simulink model "fixpt_rounding_mode"  (R2015b)
settings: Solver=FixedStepDiscrete  SolverMode=SingleTasking  StartTime=0.0  StopTime=10  RelTol=1e-3
settings Model: Creator=amatsumo  LastModifiedBy=amatsumo
settings DataIOCC: SaveFormat=Array  SignalLoggingSaveFormat=ModelDataLogs  SaveOutput=off  SignalLogging=off  SaveTime=off
settings OptimizationCC: BlockReduction=off  ConditionallyExecuteInputs=off  DefaultParameterBehavior=Inlined  ExpressionDepthLimit=2147483647
settings DebuggingCC: AlgebraicLoopMsg=error  UnderspecifiedInitializationDetection=Classic  MergeDetectMultiDrivingBlocksExec=none  SolverPrmCheckMsg=warning  SingleTaskRateTransMsg=error  FcnCallInpInsideContextMsg=EnableAllAsWarning  StateNameClashWarn=warning
settings HardwareCC: ProdBitPerPointer=32  ProdLargestAtomicFloat=None  ProdIntDivRoundTo=Undefined  ProdEndianess=Unspecified  ProdWordSize=32  ProdHWDeviceType=ASIC/FPGA->ASIC/FPGA  ProdEqTarget=off
settings GRTTargetCC: GeneratePreprocessorConditionals=Disable all  CombineOutputUpdateFcns=off  GRTInterface=on
settings ConfigComp: CovModelRefEnable=Off  CovSFcnEnable=off

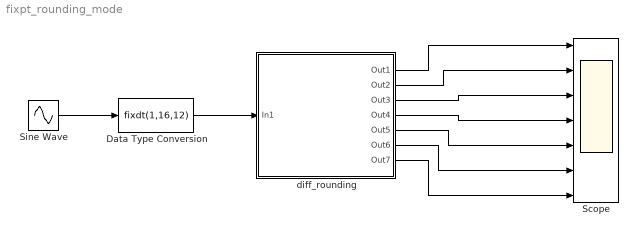
== system fixpt_rounding_mode ==
  Data Type Conversion : DataTypeConversion  OutDataTypeStr=fixdt(1,16,12)
  Scope : Scope  NumInputPorts=7
  Sine Wave : Sin  Frequency=2*pi*1  SampleTime=1/100
  diff_rounding : Subsystem
  wires:
  Sine Wave/1 -> Data Type Conversion/1
  Data Type Conversion/1 -> diff_rounding/1(In1)
  diff_rounding/1(Out1) -> Scope/1
  diff_rounding/2(Out2) -> Scope/2
  diff_rounding/3(Out3) -> Scope/3
  diff_rounding/4(Out4) -> Scope/4
  diff_rounding/5(Out5) -> Scope/5
  diff_rounding/6(Out6) -> Scope/6
  diff_rounding/7(Out7) -> Scope/7

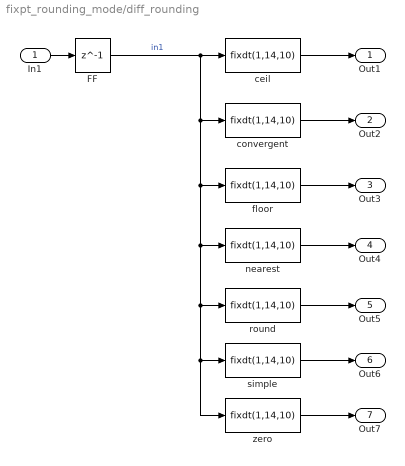
== system fixpt_rounding_mode/diff_rounding ==
  In1 : Inport
  FF : Delay  DelayLength=1
  ceil : DataTypeConversion  OutDataTypeStr=fixdt(1,14,10)  RndMeth=Ceiling
  convergent : DataTypeConversion  OutDataTypeStr=fixdt(1,14,10)  RndMeth=Convergent
  floor : DataTypeConversion  OutDataTypeStr=fixdt(1,14,10)
  nearest : DataTypeConversion  OutDataTypeStr=fixdt(1,14,10)  RndMeth=Nearest
  round : DataTypeConversion  OutDataTypeStr=fixdt(1,14,10)  RndMeth=Round
  simple : DataTypeConversion  OutDataTypeStr=fixdt(1,14,10)  RndMeth=Simplest
  zero : DataTypeConversion  OutDataTypeStr=fixdt(1,14,10)  RndMeth=Zero
  Out1 : Outport
  Out2 : Outport  Port=2
  Out3 : Outport  Port=3
  Out4 : Outport  Port=4
  Out5 : Outport  Port=5
  Out6 : Outport  Port=6
  Out7 : Outport  Port=7
  wires:
  In1/1 -> FF/1
  ceil/1 -> Out1/1
  convergent/1 -> Out2/1
  floor/1 -> Out3/1
  nearest/1 -> Out4/1
  round/1 -> Out5/1
  simple/1 -> Out6/1
  zero/1 -> Out7/1
  FF/1 -> zero/1, simple/1, round/1, nearest/1, floor/1, convergent/1, ceil/1  "in1"
